simulink model "sim_continuo_vs_discreto_control_integral_observador_simple"  (R2016a)
settings: Solver=VariableStepAuto  StartTime=0.0  StopTime=0.2  RelTol=1e-5
values from neighbouring files (symbols this model uses):
  A = [0 1 ... (first row only)    [calculate_gains.m]    (also in get_linear_model.m = jacobian(xp_nl,x_state))
  B = [0 ... (first row only)    [calculate_gains.m]    (also in get_linear_model.m = jacobian(xp_nl,u_state))
  C = [1 0]    [calculate_gains.m]    (also in get_linear_model.m = jacobian(y_nl,x_state))
  Kdi = calc_discrete_integral_controller_gains(A,B,C,Pi,Ts)    [generate_lookup_table.m]
  Ki = calc_integral_controller_gains(A,B,C,Pi)    [generate_lookup_table.m]
  Ts = 4e-4    (= 0.0004)    [calculate_gains.m]    (also in generate_lookup_table.m = 0.0005)
undefined symbols (not defined in the file or in its folder): Ad, Bd, Cd, DiscIntNeverNeededParam, Kdo, Ko
settings Model: Creator=manuel  LastModifiedBy=manuel

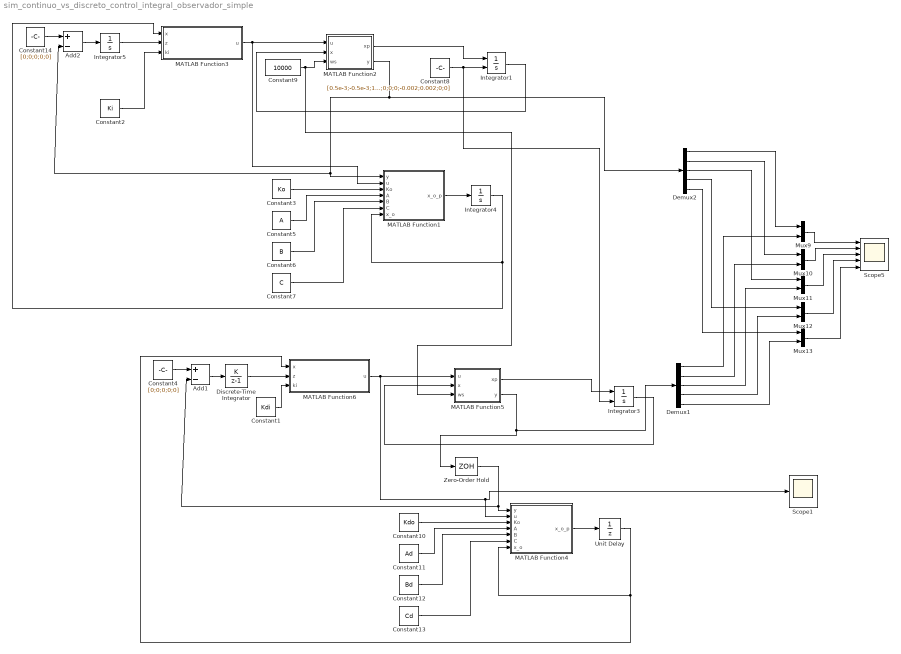
== system sim_continuo_vs_discreto_control_integral_observador_simple ==
  Add1 : Sum  Inputs=+-
  Add2 : Sum  Inputs=+-
  Constant1 : Constant  Value=Kdi  VectorParams1D=off
  Constant10 : Constant  Value=Kdo  VectorParams1D=off
  Constant11 : Constant  Value=Ad  VectorParams1D=off
  Constant12 : Constant  Value=Bd  VectorParams1D=off
  Constant13 : Constant  Value=Cd  VectorParams1D=off
  Constant14 : Constant  Value=[0;0;0;0;0]
  Constant2 : Constant  Value=Ki  VectorParams1D=off
  Constant3 : Constant  Value=Ko  VectorParams1D=off
  Constant4 : Constant  Value=[0;0;0;0;0]
  Constant5 : Constant  Value=A  VectorParams1D=off
  Constant6 : Constant  Value=B  VectorParams1D=off
  Constant7 : Constant  Value=C  VectorParams1D=off
  Constant8 : Constant  Value=[0.5e-3;-0.5e-3;1e-3;0;0;0;-0.002;0.002;0;0]
  Constant9 : Constant  Value=10000  VectorParams1D=off
  Demux1 : Demux  Outputs=5
  Demux2 : Demux  Outputs=5
  Discrete-Time Integrator : DiscreteIntegrator  IntegratorMethod=Accumulation: Forward Euler  gainval=1  InitialCondition=[0;0;0;0;0]  InitialConditionSetting=State (most efficient)  SampleTime=-1  ICPrevOutput=DiscIntNeverNeededParam  ICPrevScaledInput=DiscIntNeverNeededParam
  Integrator1 : Integrator  InitialConditionSource=external  InitialCondition=[0;0;0;0;0;0;0;0;0;0]
  Integrator3 : Integrator  InitialConditionSource=external  InitialCondition=[0;0;0;0;0;0;0;0;0;0]
  Integrator4 : Integrator  InitialCondition=[0;0;0;0;0;0;0;0;0;0]
  Integrator5 : Integrator  InitialCondition=[0;0;0;0;0]
  MATLAB Function1 : MATLAB Function  TreatAsAtomicUnit=on
  MATLAB Function2 : MATLAB Function  TreatAsAtomicUnit=on
  MATLAB Function3 : MATLAB Function  TreatAsAtomicUnit=on
  MATLAB Function4 : MATLAB Function  TreatAsAtomicUnit=on
  MATLAB Function5 : MATLAB Function  TreatAsAtomicUnit=on
  MATLAB Function6 : MATLAB Function  TreatAsAtomicUnit=on
  Mux{9..13} (5 alike) : Mux  Inputs=2
  Scope1 : Scope
  Scope5 : Scope  NumInputPorts=5
  Unit Delay : UnitDelay  InitialCondition=[0;0;0;0;0;0;0;0;0;0]  SampleTime=-1
  Zero-Order Hold : ZeroOrderHold  SampleTime=Ts
  wires:
  Integrator3/1 -> MATLAB Function5/2(x)
  Add1/1 -> Discrete-Time Integrator/1
  MATLAB Function5/1(xp) -> Integrator3/1
  MATLAB Function5/2(y) -> Zero-Order Hold/1, Demux1/1
  MATLAB Function4/1(x_o_p) -> Unit Delay/1
  Constant10/1 -> MATLAB Function4/3(Ko)
  Constant11/1 -> MATLAB Function4/4(A)
  Constant12/1 -> MATLAB Function4/5(B)
  Constant13/1 -> MATLAB Function4/6(C)
  Unit Delay/1 -> MATLAB Function4/7(x_o), MATLAB Function6/1(x)
  MATLAB Function6/1(u) -> MATLAB Function5/1(u), Scope1/1, MATLAB Function4/2(u)
  Mux9/1 -> Scope5/1
  Mux10/1 -> Scope5/2
  Mux11/1 -> Scope5/3
  Mux12/1 -> Scope5/4
  Mux13/1 -> Scope5/5
  Demux1/2 -> Mux10/2
  Demux1/1 -> Mux9/2
  Demux1/3 -> Mux11/2
  Demux1/4 -> Mux12/2
  Demux1/5 -> Mux13/2
  Demux2/1 -> Mux9/1
  Demux2/2 -> Mux10/1
  Demux2/3 -> Mux11/1
  Demux2/4 -> Mux12/1
  Demux2/5 -> Mux13/1
  Constant1/1 -> MATLAB Function6/3(ki)
  Zero-Order Hold/1 -> Add1/2, MATLAB Function4/1(y)
  Constant4/1 -> Add1/1
  Discrete-Time Integrator/1 -> MATLAB Function6/2(z)
  Integrator1/1 -> MATLAB Function2/2(x)
  Add2/1 -> Integrator5/1
  MATLAB Function2/1(xp) -> Integrator1/1
  MATLAB Function1/1(x_o_p) -> Integrator4/1
  Constant3/1 -> MATLAB Function1/3(Ko)
  Constant5/1 -> MATLAB Function1/4(A)
  Constant6/1 -> MATLAB Function1/5(B)
  Constant7/1 -> MATLAB Function1/6(C)
  Integrator4/1 -> MATLAB Function1/7(x_o), MATLAB Function3/1(x)
  MATLAB Function3/1(u) -> MATLAB Function2/1(u), MATLAB Function1/2(u)
  Constant2/1 -> MATLAB Function3/3(ki)
  MATLAB Function2/2(y) -> MATLAB Function1/1(y), Add2/2, Demux2/1
  Constant14/1 -> Add2/1
  Integrator5/1 -> MATLAB Function3/2(z)
  Constant9/1 -> MATLAB Function5/3(ws), MATLAB Function2/3(ws)
  Constant8/1 -> Integrator3/2, Integrator1/2

== matlab function sim_continuo_vs_discreto_control_integral_observador_simple/MATLAB Function1 ==
  data: y input; u input; x_o_p output; Ko input; A input; B input; C input; x_o input
function x_o_p = state_obsever(y,u,Ko,A,B,C,x_o)
%#codegen
x_o_p = A*x_o + B*u + Ko*(y-C*x_o);

== matlab function sim_continuo_vs_discreto_control_integral_observador_simple/MATLAB Function4 ==
  data: y input; u input; x_o_p output; Ko input; A input; B input; C input; x_o input
function x_o_p = state_obsever(y,u,Ko,A,B,C,x_o)
%#codegen
x_o_p = A*x_o + B*u + Ko*(y-C*x_o);

== matlab function sim_continuo_vs_discreto_control_integral_observador_simple/MATLAB Function2 ==
  data: u input; x input; xp output; y output; ws input
function [xp,y] = fcn(u,x,ws)

Fd_x = 0;
Fd_y = 0;
Fd_z = 0;
Md_y = 0;
Md_z = 0;
Fmcce1 = 0;
Fmcce2 = 0;
[xp,y] = hmb_non_linear_model(x,u,ws,Fd_x,Fd_y,Fd_z,Md_y,Md_z,Fmcce1,Fmcce2);
end

== matlab function sim_continuo_vs_discreto_control_integral_observador_simple/MATLAB Function3 ==
  data: x input; z input; u output; ki input
function u  = integral_controller(x,z,ki)
%#codegen
xi = [x;z];
u = -ki*xi;

== matlab function sim_continuo_vs_discreto_control_integral_observador_simple/MATLAB Function5 ==
  data: u input; x input; xp output; y output; ws input
function [xp,y] = fcn(u,x,ws)

Fd_x = 0;
Fd_y = 0;
Fd_z = 0;
Md_y = 0;
Md_z = 0;
Fmcce1 = 0;
Fmcce2 = 0;
[xp,y] = hmb_non_linear_model(x,u,ws,Fd_x,Fd_y,Fd_z,Md_y,Md_z,Fmcce1,Fmcce2);
end

== matlab function sim_continuo_vs_discreto_control_integral_observador_simple/MATLAB Function6 ==
  data: x input; z input; u output; ki input
function u  = integral_controller(x,z,ki)
%#codegen
xi = [x;z];
u = -ki*xi;
